simulink model "FourWheelSim_base"  (R2021b)
settings: Solver=ode4  StartTime=0.0  StopTime=100  FixedStep=0.001  EnableMultiTasking=on
values from neighbouring files (symbols this model uses):
  a_f = [1.434106444513048,-3.490394354141787e-04,2.761516722659314,6.000050177239062e+04,2.990012596710455e+03,-1.736376596503330e-04,0.526021936511837]    [VehicleParams20_ver230707.m]
  a_r = a_f    [VehicleParams20_ver230707.m]
  afx_f = [1.736519934348130,-2.903281841026900e-04,2.651682004580759,7.000047010028531e+04,3.270011055825476e+03,-0.001252141095807,1.596836353939939]    [VehicleParams20_ver230707.m]
  afx_r = afx_f    [VehicleParams20_ver230707.m]
  agx_f = [0.230000000000000,2.936116597489246e+04,7.137436879966481e+03,0,0]    [VehicleParams20_ver230707.m]
  agx_r = agx_f    [VehicleParams20_ver230707.m]
  agy_f = [0.852564208514954,3.000069064154418e+04,2.070023877794581e+03,-5.089267464508360e-04,0.519364283925805]    [VehicleParams20_ver230707.m]
  agy_r = agy_f    [VehicleParams20_ver230707.m]
  b_f = [3.436650779629654,1.566044221042620e-05,0.028598122547093,3.408741969645286e+03,5.995144285148312e+03,-1.736376595720277e-04,0.526021936449385]    [VehicleParams20_ver230707.m]
  Brake_Factor = 0.66    [VehicleParams20_ver230707.m]
  Cd = Cd/(40/3.6)^2    (= 0.6885)    [VehicleParams20_ver230707.m]
  CLF = DFf/40/40    (= 0.06)    [VehicleParams20_ver230707.m]
  CLR = DFr/40/40    (= 0.065)    [VehicleParams20_ver230707.m]
  cPiston_Area_F = 2*pi*(0.0254/2)^2    (= 0.00101341495819)    [VehicleParams20_ver230707.m]
  cPiston_Area_R = 2*pi*(0.0254/2)^2    (= 0.00101341495819)    [VehicleParams20_ver230707.m]
  delta = 15.5    [VehicleParams20_ver230707.m]
  df = 1.225    [VehicleParams20_ver230707.m]
  dr = 1.225    [VehicleParams20_ver230707.m]
  eff_Radius_F = (180/2-13.5)/1000    (= 0.0765)    [VehicleParams20_ver230707.m]
  eff_Radius_R = (180/2-13.5)/1000    (= 0.0765)    [VehicleParams20_ver230707.m]
  Fd = 60*2    (= 120)    [VehicleParams20_ver230707.m]
  Frtoe = 0    [VehicleParams20_ver230707.m]
  gear_f = 13.75    [VehicleParams20_ver230707.m]
  gear_r = 13.75    [VehicleParams20_ver230707.m]
  hg = 0.28    [VehicleParams20_ver230707.m]
  HV_voltage = 600    [VehicleParams20_ver230707.m]
  I = 112    [VehicleParams20_ver230707.m]
  ini_v = ini_speed/3.6    (= 10.4166666667)    [VehicleParams20_ver230707.m]
  Kframe = 5.94*10^6    (= 5940000)    [VehicleParams20_ver230707.m]
  kk_f = 2800*180/pi    (= 160428.182637)    [VehicleParams20_ver230707.m]
  kk_r = 4200*180/pi    (= 240642.273955)    [VehicleParams20_ver230707.m]
  krfr = 0.5    [VehicleParams20_ver230707.m]
  l = 1.530    (= 1.53)    [VehicleParams20_ver230707.m]
  lf = l*(1-WBf)    (= 0.7956)    [VehicleParams20_ver230707.m]
  lr = l*WBf    (= 0.7344)    [VehicleParams20_ver230707.m]
  M = 200+60    (= 260)    [VehicleParams20_ver230707.m]
  mu_tire_F = 0.587-0.587+0.55    (= 0.55)    [VehicleParams20_ver230707.m]
  mu_tire_R = 0.587-0.587+0.55    (= 0.55)    [VehicleParams20_ver230707.m]
  Mwf = Iwf/Rwf/Rwf    (= 3.82716814816)    [VehicleParams20_ver230707.m]
  Mwr = Iwr/Rwr/Rwr    (= 3.82716814816)    [VehicleParams20_ver230707.m]
  rcf = 0.000    (= 0)    [VehicleParams20_ver230707.m]
  rch = rcf*WBf+rcr*(1-WBf)    (= 0)    [VehicleParams20_ver230707.m]
  rcr = 0.000    (= 0)    [VehicleParams20_ver230707.m]
  Reartoe = -2    [VehicleParams20_ver230707.m]
  Rr_toe = Reartoe*pi/180    (= -0.0349065850399)    [VehicleParams20_ver230707.m]
  Rwf = 18*(25.4/1000)/2    (= 0.2286)    [VehicleParams20_ver230707.m]
  Rwr = 18*(25.4/1000)/2    (= 0.2286)    [VehicleParams20_ver230707.m]
  T_TireF = TireL_f/V    (= 0.036760000032)    [VehicleParams20_ver230707.m]
  T_TireR = TireL_r/V    (= 0.036760000032)    [VehicleParams20_ver230707.m]
  tspeed = 37.5    [VehicleParams20_ver230707.m]
  WBf = 0.48    [VehicleParams20_ver230707.m]
  zc_f = castrail_Fr/1000    (= 0)    [VehicleParams20_ver230707.m]
  zc_r = castrail_Rr/1000    (= 0)    [VehicleParams20_ver230707.m]
libraries: simulink x25, dspstat3 x1
(part 1 of 4)
settings Model: Creator=FEM  LastModifiedBy=tsuyoshi
settings SolverCC: ZeroCrossAlgorithm=Adaptive  AlgebraicLoopSolver=TrustRegion
settings DataIOCC: LimitDataPoints=on  SaveFormat=Array  ReturnWorkspaceOutputs=off
settings OptimizationCC: ExpressionDepthLimit=2147483647  LifeSpan=inf
settings DebuggingCC: UnderspecifiedInitializationDetection=Classic  MergeDetectMultiDrivingBlocksExec=none  MaxConsecutiveZCsMsg=none  SolverPrmCheckMsg=warning  StateNameClashWarn=warning  SFUnexpectedBacktrackingDiag=warning  SFNoUnconditionalDefaultTransitionDiag=warning  SFExecutionAtInitializationDiag=none  SFMachineParentedDataDiag=warning  ArithmeticOperatorsInVariantConditions=warning
settings HardwareCC: ProdBitPerPointer=32  ProdBitPerSizeT=32  ProdBitPerPtrDiffT=32  ProdLargestAtomicFloat=None  ProdIntDivRoundTo=Undefined  ProdEndianess=Unspecified  ProdWordSize=32  ProdHWDeviceType=32-bit Generic
settings ModelReferenceCC: PropagateSignalLabelsOutOfModel=off
settings SFSimCC: SimUseLocalCustomCode=off  CustomCodeUndefinedFunction=UseInterfaceOnly
settings RTWCC: RTWUseLocalCustomCode=off
settings CodeAppCC: StateflowObjectComments=on
settings GRTTargetCC: TargetLangStandard=C89/C90 (ANSI)
settings ConfigComp: CovMetricSettings=dw  CovSaveCumulativeToWorkspaceVar=on  CovSaveSingleToWorkspaceVar=on  CovExternalEMLEnable=off
settings SimscapeCC: SimscapeNormalizeSystem=off

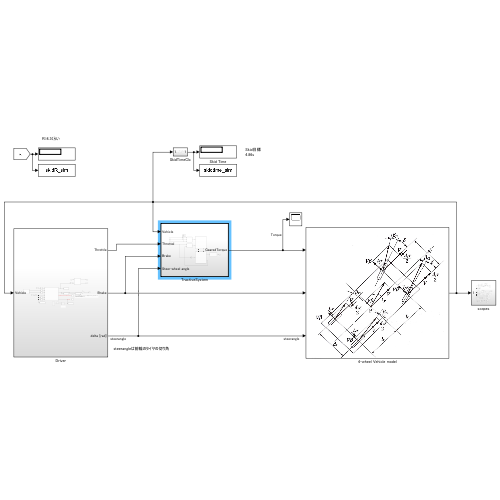
[thumbnail: Simulink's stored preview of the top-level diagram]
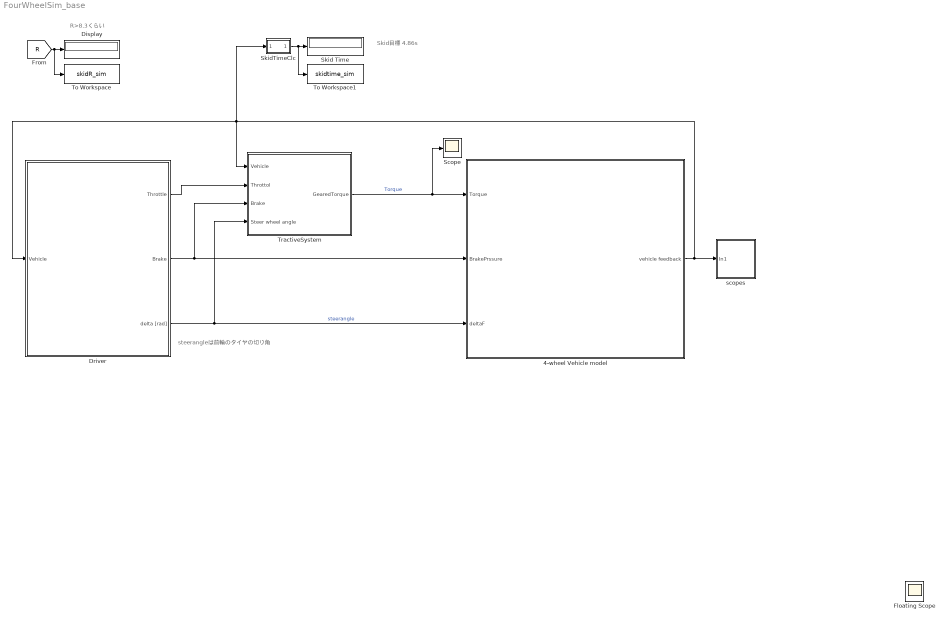
== system FourWheelSim_base ==
  note: R>8.3くらい
  note: Skid目標
      | 4.86s
  note: steerangleは前輪のタイヤの切り角
  4-wheel Vehicle model : Subsystem
      mask Display: image('$imagefile'); % 変更するには、ツールストリップの [イメージの編集] を使用してください。
  Display : Display
  Driver : Subsystem
  Scope : Scope
  Skid Time : Display
  SkidTimeClc : Subsystem
  To Workspace : ToWorkspace  VariableName=skidR_sim  SaveFormat=Timeseries  SampleTime=-1
  To Workspace1 : ToWorkspace  VariableName=skidtime_sim  SaveFormat=Timeseries  SampleTime=-1
  TractiveSystem : Subsystem  TreatAsAtomicUnit=on
  scopes : Subsystem
  Floating Scope : Scope
  wires:
  Driver/1(Throttle) -> TractiveSystem/2(Throttol)
  TractiveSystem/1(GearedTorque) -> 4-wheel Vehicle model/1(Torque), Scope/1  "Torque"
  4-wheel Vehicle model/1(vehicle feedback) -> SkidTimeClc/1(In1), Driver/1(Vehicle), TractiveSystem/1(Vehicle), scopes/1(In1)
  SkidTimeClc/1(Out1) -> To Workspace1/1, Skid Time/1
  [R] -> To Workspace/1, Display/1
  Driver/2(Brake) -> 4-wheel Vehicle model/2(BrakePrssure), TractiveSystem/3(Brake)
  Driver/3(delta [rad]) -> TractiveSystem/4(Steer wheel angle), 4-wheel Vehicle model/3(deltaF)  "steerangle"

== system FourWheelSim_base/4-wheel Vehicle model ==
  Torque : Inport
  BrakePrssure : Inport  Port=2
  deltaF : Inport  Port=3
  BrakeSystem : Subsystem
  Bus Creator2 : BusCreator  Inputs=4
  Constant : Constant  Value=Rr_toe
  Fin : Fcn  Expr=u+Frtoe*pi/180
  Fout : Fcn  Expr=u-Frtoe*pi/180
  Gain7 : Gain  Gain=-1
  comb slip model : Subsystem
      mask Display: image('$imagefile'); % 変更するには、ツールストリップの [イメージの編集] を使用してください。
  "equation of motion " : Subsystem
      mask Display: image('$imagefile'); % 変更するには、ツールストリップの [イメージの編集] を使用してください。
  force direction change : Subsystem
  to workspace : Subsystem
  vehicle feedback : Outport  VectorParamsAs1DForOutWhenUnconnected=off
  wires:
  Constant/1 -> Gain7/1, Bus Creator2/3  "delta_RL"
  comb slip model/1(tire force) -> force direction change/1(tire force)  "tire force"
  Bus Creator2/1 -> comb slip model/3(delta), force direction change/2(delta)  "delta"
  deltaF/1 -> Fin/1, Fout/1
  "equation of motion "/1(Vehicle Motion) -> to workspace/1(In1), comb slip model/1(Vehicle Motion)  "Vehicle Motion"
  Fout/1 -> Bus Creator2/2  "delta_FR"
  Fin/1 -> Bus Creator2/1  "delta_FL"
  Gain7/1 -> Bus Creator2/4  "delta_RR"
  Torque/1 -> BrakeSystem/2(GearedTorque)
  comb slip model/2(vehicle feedback) -> vehicle feedback/1
  force direction change/1(Long Force) -> "equation of motion "/1(Long Force)  "Long Force"
  force direction change/2(Yaw Moment) -> "equation of motion "/2(Yaw Moment)  "Yaw Moment"
  force direction change/3(Lat Force) -> "equation of motion "/3(Lat Force)  "Lat Force"
  BrakePrssure/1 -> BrakeSystem/1(BrakePrssure)
  BrakeSystem/1(NetTorque) -> comb slip model/2(Torque)

== system FourWheelSim_base/Driver ==
  note: 発散の原因
      | DYCゲイン過大：1
      | その他(トー過大?)：2
  note: Goto/Fromでつないだ場合，
      | 「Goto/From の接続は、非バーチャル サブシステムの境界をクロスできません。唯一の例外は、Goto が状態出力端子に接続される場合のみです」
      | エラーとなるのでForループを用いる．
  Vehicle : Inport
  Chart : Stateflow chart  TreatAsAtomicUnit=on
  Constant1 : Constant  Commented=on  Value=2
  Display : Display
  Gain1 : Gain  Gain=pi/180
  Memory{,1..3} (4 alike) : Memory
  Pylon Touch : Subsystem
  Saturation : Saturate  UpperLimit=200  LowerLimit=0
  SpeedControll : Subsystem
  Stop Simulation : Stop
  Stop Simulation1 : Stop
  Switch1 : Switch  Commented=on  Threshold=340*pi/360
  To Workspace1 : ToWorkspace  VariableName=Div  SaveFormat=Timeseries  SampleTime=-1
  To Workspace2 : ToWorkspace  VariableName=tspeed_sim  SaveFormat=Timeseries  SampleTime=-1
  To Workspace3 : ToWorkspace  VariableName=delta_sim  SaveFormat=Timeseries  SampleTime=-1
  To Workspace4 : ToWorkspace  VariableName=Vnow_sim  SaveFormat=Timeseries  SampleTime=-1
  Transport Delay : TransportDelay
  Transport Delay1 : TransportDelay  DelayTime=0.5
  βの最大変化量 : Subsystem  Commented=on
  Throttle : Outport
  Brake : Outport  Port=2
  delta [rad] : Outport  Port=3
  wires:
  Transport Delay/1 -> Chart/5(Vpre1)
  Pylon Touch/1(Rf) -> Memory1/1
  Pylon Touch/2(Rr) -> Memory2/1
  Chart/2(delta) -> To Workspace3/1, Gain1/1, Display/1
  [R] -> Memory/1
  Chart/3(Vopt) -> ?
  Chart/4(Div) -> To Workspace1/1
  Memory/1 -> Chart/1(R)
  Memory1/1 -> Chart/2(Rf)
  Memory2/1 -> Chart/3(Rr)
  [Vnow] -> Memory3/1
  Memory3/1 -> Transport Delay/1, To Workspace4/1, Transport Delay1/1, Chart/4(Vnow)
  Constant1/1 -> Switch1/1
  βの最大変化量/1(Outport) -> Switch1/2
  Transport Delay1/1 -> Chart/6(Vpre05)
  Saturation/1 -> SpeedControll/2(Target Speed)
  Chart/1(tspeed) -> Saturation/1, To Workspace2/1  "TargetSpeed(km/h)"
  Vehicle/1 -> SpeedControll/1(Vehicle speed)
  SpeedControll/1(Throttle) -> Throttle/1
  SpeedControll/2(Brake) -> Brake/1
  Gain1/1 -> delta [rad]/1  "deltaF(rad)"

== system FourWheelSim_base/SkidTimeClc ==
  In1 : Inport
  Bus Selector : BusSelector  OutputSignals=Vehicle Motion.Long Velocity
  Divide : Product  Inputs=*/
  Gain : Gain  Gain=2*pi
  m/s : Gain
  Out1 : Outport  VectorParamsAs1DForOutWhenUnconnected=off
  wires:
  m/s/1 -> Divide/2
  In1/1 -> Bus Selector/1
  [R] -> Gain/1
  Divide/1 -> Out1/1
  Gain/1 -> Divide/1
  Bus Selector/1 -> m/s/1  "<Long Velocity>"

== system FourWheelSim_base/TractiveSystem ==
  Vehicle : Inport
  Throttol : Inport  Port=2
  Brake : Inport  Port=3
  Steer wheel angle : Inport  Port=4
  AMK PowerUnit x4 : Subsystem
      settings: PortSchema="{\"entries\":[{\"content\":{\"sides\":[{\"content\":{\"connectorIds\":[\"In1\"]},\"type\":\"ConnectorPlacement.EquallySpacedRectSide\",\"uuid\":\"e990d11b-ff81-4335-9a22-6cdf713d4717\"},{\"content\":{\"connectorIds\":[\"Out1\",\"Out2\"],\"side\":\"RIGHT\"},\"type\":\"ConnectorPlacement.EquallySpacedRectSide\",\"uuid\":\"59e0e618-bfe7-45fe-904d-89bd6da9458c\"},{\"content\":{\"connectorIds\":[\"Out3\",\"In2\"],\"side\":\"TOP\"},\"type\":\"ConnectorPlacement.EquallySpacedRectSide\",\"uuid\":\"9e2b5955-7a03-4a6a-9f05-18476f3458b2\"}]},\"type\":\"ConnectorPlacement.EquallySpacedConnector\",\"uuid\":\"65fbb8fc-573a-4a64-b281-fb493310408d\"}],\"packageUris\":[\"http://schema.mathworks.com/mf0/Connector/R2020b\"],\"version\":\"1.0\"}"
  Bus Selector1 : BusSelector  OutputSignals=Wheel Speed
  Driver Input : Subsystem
  Gear : Subsystem
  Scope : Scope  NumInputPorts=3
  Sensors : Subsystem
  VCM : Subsystem
      settings: PortSchema="{\"entries\":[{\"content\":{\"sides\":[{\"content\":{\"connectorIds\":[\"In1\",\"In2\"]},\"type\":\"ConnectorPlacement.EquallySpacedRectSide\",\"uuid\":\"5e77dd93-b51c-479b-b5fe-6f6816a8f554\"},{\"content\":{\"connectorIds\":[],\"side\":\"RIGHT\"},\"type\":\"ConnectorPlacement.EquallySpacedRectSide\",\"uuid\":\"bf0d52ae-9b9e-4d5a-babc-26efa99ef7a4\"},{\"content\":{\"connectorIds\":[],\"side\":\"TOP\"},\"type\":\"ConnectorPlacement.EquallySpacedRectSide\",\"uuid\":\"b9d2ff59-7c1f-4a33-8b92-e641dfa19e52\"},{\"content\":{\"connectorIds\":[\"In3\",\"Out1\"],\"side\":\"BOTTOM\"},\"type\":\"ConnectorPlacement.EquallySpacedRectSide\",\"uuid\":\"e471c7ad-4e4d-4a43-b287-ecb0303bfc1b\"}]},\"type\":\"ConnectorPlacement.EquallySpacedConnector\",\"uuid\":\"5754af0f-8218-4685-b773-d9359332d734\"}],\"packageUris\":[\"http://schema.mathworks.com/mf0/Connector/R2020b\"],\"version\":\"1.0\"}"
  GearedTorque : Outport  VectorParamsAs1DForOutWhenUnconnected=off
  wires:
  Bus Selector1/1 -> AMK PowerUnit x4/1(Wheel speed)  "<Wheel Speed>"
  VCM/1(CAN out) -> AMK PowerUnit x4/2(CAN in)
  Driver Input/1(Driver Input) -> VCM/1(Driver in)
  AMK PowerUnit x4/3(CAN out) -> VCM/3(CAN in)
  Sensors/1(CAN to VCM) -> VCM/2(Sensor)
  AMK PowerUnit x4/2(Current) -> Sensors/2(Current)
  Throttol/1 -> Scope/1, Driver Input/1(Throttol)
  Vehicle/1 -> Bus Selector1/1, Sensors/1(Sensors)
  Steer wheel angle/1 -> Scope/3, Driver Input/3(Steer angle)
  Gear/1(GearedTorque) -> GearedTorque/1
  AMK PowerUnit x4/1(Motor trq) -> Gear/1(MotorTorque)
  Brake/1 -> Scope/2, Driver Input/2(Brake)

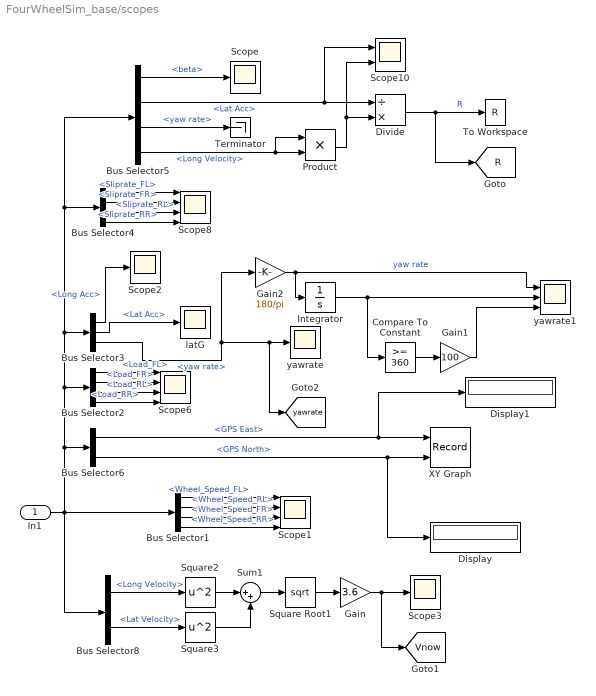
== system FourWheelSim_base/scopes ==
  In1 : Inport
  Bus Selector1 : BusSelector  OutputSignals=Wheel Speed.Wheel_Speed_FL,Wheel Speed.Wheel_Speed_RL,Wheel Speed.Wheel_Speed_FR,Wheel Speed.Wheel_Speed_RR
  Bus Selector2 : BusSelector  OutputSignals=tire status.load.Load_FL,tire status.load.Load_FR,tire status.load.Load_RL,tire status.load.Load_RR
  Bus Selector3 : BusSelector  OutputSignals=Vehicle Motion.Long Acc,Vehicle Motion.Lat Acc,Vehicle Motion.yaw rate
  Bus Selector4 : BusSelector  OutputSignals=tire status.Slip rate.Sliprate_FL,tire status.Slip rate.Sliprate_FR,tire status.Slip rate.Sliprate_RL,tire status.Slip rate.Sliprate_RR
  Bus Selector5 : BusSelector  OutputSignals=Vehicle Motion.beta,Vehicle Motion.Lat Acc,Vehicle Motion.yaw rate,Vehicle Motion.Long Velocity
  Bus Selector6 : BusSelector  OutputSignals=Vehicle Motion.GPS East,Vehicle Motion.GPS North
  Bus Selector8 : BusSelector  OutputSignals=Vehicle Motion.Long Velocity,Vehicle Motion.Lat Velocity
  Compare To Constant : simulink/Logic and Bit Operations/Compare To Constant  relop=>=  const=360  OutDataTypeStr=boolean
  Display : Display
  Display1 : Display
  Divide : Product  Inputs=/*
  Gain : Gain  Gain=3.6
  Gain1 : Gain  Gain=100
  Gain2 : Gain  Gain=180/pi
  Integrator : Integrator
  Product : Product
  Scope : Scope
  Scope1 : Scope  NumInputPorts=4
  Scope10 : Scope  NumInputPorts=2
  Scope2 : Scope
  Scope3 : Scope
  Scope6 : Scope  NumInputPorts=4
  Scope8 : Scope  NumInputPorts=4
  Square Root1 : Sqrt  SaturateOnIntegerOverflow=on
  Square2 : Math  Operator=square  SaturateOnIntegerOverflow=on
  Square3 : Math  Operator=square  SaturateOnIntegerOverflow=on
  Sum1 : Sum  Inputs=|++
  Terminator : Terminator
  To Workspace : ToWorkspace  VariableName=R  SaveFormat=Timeseries  SampleTime=-1
  XY Graph : Record  FileSettingsInternal="{\"entries\":[{\"content\":{\"excelSettings\":{\"content\":{},\"type\":\"Streamout.ExcelSettings\"}},\"type\":\"Streamout.FileSettingStorage\",\"uuid\":\"04da413e-0bc8-4522-bc77-97f7bd740fff\"}],\"packageUris\":[\"http://schema.mathworks.com/mf0/streamout_blocks/R2020a\"],\"version\":\"1.0\"}"  Layout=[1 1]  SignalsInternal="{\"entries\":[{\"content\":{\"signals\":[{\"content\":{\"blockPath\":[\"FourWheelSim_base/scopes/XY Graph\"],\"channel\":[],\"dimensions\":[1],\"domain\":\"FourWheelSim_base/scopes/XY Graph\",\"lineColor\":\"#77ac30\",\"plots\":[1],\"port\":1,\"sid\":[],\"signalID\":713,\"signalName\":\"<GPS East>\"},\"type\":\"RecordBlkView.Signal\",\"uuid\":\"76456aae-c6a4-477c-b0e6-9aa2acff60b4\"},{\"content\":{\"blockPath\":[\"FourWheelSim_base/scopes/XY Graph\"],\"channel\":[],\"dimensions\":[1],\"domain\":\"FourWheelSim_base/scopes/XY Graph\",\"lineColor\":\"#4dbeee\",\"plots\":[1],\"port\":2,\"sid\":[],\"signalID\":716,\"signalName\":\"<GPS North>\"},\"type\":\"RecordBlkView.Signal\",\"uuid\":\"c308d40b-e731-4fe8-a725-c3bc60c488fc\"}]},\"type\":\"RecordBlkView.InputSignals\",\"uuid\":\"f0e00ebc-5757-4aa9-ad1b-0663875eda47\"}],\"packageUris\":[\"http://schema.mathworks.com/mf0/streamout_blocks/R2020a\"],\"version\":\"1.0\"}"  VisualizationBindings="{\"xyplotplugin\":{\"info\":[{\"series\":[{\"bindingParametersList\":[{\"parameter\":\"X-Axis\",\"signalID\":713,\"signalName\":\"<GPS East>\"},{\"parameter\":\"Y-Axis\",\"signalID\":716,\"signalName\":\"<GPS North>\"}],\"seriesID\":50809}],\"subplotID\":1}]}}"  CompatibilityTag=XY  st=-1
  latG : Scope
  yawrate : Scope
  yawrate1 : Scope  NumInputPorts=3
  tag scope: R=global, Vnow=global, yawrate=global
  wires:
  Bus Selector3/2 -> latG/1  "<Lat Acc>"
  Compare To Constant/1 -> Gain1/1
  Bus Selector2/2 -> Scope6/2  "<Load_FR>"
  Gain2/1 -> Integrator/1, yawrate1/1  "yaw rate"
  Bus Selector5/1 -> Scope/1  "<beta>"
  Product/1 -> Divide/2, Scope10/2
  Divide/1 -> To Workspace/1, [R]  "R"
  Gain1/1 -> yawrate1/3
  Bus Selector4/1 -> Scope8/1  "<Sliprate_FL>"
  Bus Selector5/4 -> Product/1, Product/2  "<Long Velocity>"
  Bus Selector2/3 -> Scope6/3  "<Load_RL>"
  Bus Selector2/4 -> Scope6/4  "<Load_RR>"
  Bus Selector4/2 -> Scope8/2  "<Sliprate_FR>"
  Bus Selector4/3 -> Scope8/3  "<Sliprate_RL>"
  Bus Selector4/4 -> Scope8/4  "<Sliprate_RR>"
  Bus Selector3/3 -> [yawrate], yawrate/1, Gain2/1  "<yaw rate>"
  Bus Selector5/2 -> Scope10/1, Divide/1  "<Lat Acc>"
  Integrator/1 -> Compare To Constant/1, yawrate1/2
  Bus Selector2/1 -> Scope6/1  "<Load_FL>"
  Bus Selector5/3 -> Terminator/1  "<yaw rate>"
  Bus Selector1/1 -> Scope1/1  "<Wheel_Speed_FL>"
  Bus Selector1/2 -> Scope1/2  "<Wheel_Speed_RL>"
  Bus Selector1/3 -> Scope1/3  "<Wheel_Speed_FR>"
  Bus Selector1/4 -> Scope1/4  "<Wheel_Speed_RR>"
  Bus Selector6/1 -> Display1/1, XY Graph/1  "<GPS East>"
  Bus Selector6/2 -> Display/1, XY Graph/2  "<GPS North>"
  Square Root1/1 -> Gain/1
  Square3/1 -> Sum1/2
  Bus Selector8/2 -> Square3/1  "<Lat Velocity>"
  Bus Selector8/1 -> Square2/1  "<Long Velocity>"
  Square2/1 -> Sum1/1
  Gain/1 -> [Vnow], Scope3/1
  Sum1/1 -> Square Root1/1
  In1/1 -> Bus Selector8/1, Bus Selector6/1, Bus Selector5/1, Bus Selector4/1, Bus Selector3/1, Bus Selector2/1, Bus Selector1/1
  Bus Selector3/1 -> Scope2/1  "<Long Acc>"

== system FourWheelSim_base/4-wheel Vehicle model/BrakeSystem ==
  BrakePrssure : Inport
  GearedTorque : Inport  Port=2
  Add{,1..3} (4 alike) : Sum  Inputs=+-
  Bus Creator : BusCreator  Inputs=4
  Bus Selector : BusSelector  OutputSignals=FL,FR,RL,RR
  Gain2 : Gain  Gain=cPiston_Area_F*Brake_Factor*eff_Radius_F
  Gain4 : Gain  Gain=cPiston_Area_R*Brake_Factor*eff_Radius_R
  NetTorque : Outport  VectorParamsAs1DForOutWhenUnconnected=off
  wires:
  Bus Selector/2 -> Add1/1  "<FR>"
  Gain2/1 -> Add1/2, Add/2  "BrakeTorqueFr"
  Add2/1 -> Bus Creator/3  "RL"
  Add/1 -> Bus Creator/1  "FL"
  BrakePrssure/1 -> Gain4/1, Gain2/1
  Bus Selector/3 -> Add2/1  "<RL>"
  Bus Selector/1 -> Add/1  "<FL>"
  Bus Selector/4 -> Add3/1  "<RR>"
  Gain4/1 -> Add3/2, Add2/2  "BrakeTorqueRr"
  Bus Creator/1 -> NetTorque/1  "NetTorque"
  GearedTorque/1 -> Bus Selector/1
  Add1/1 -> Bus Creator/2  "FR"
  Add3/1 -> Bus Creator/4  "RR"

== system FourWheelSim_base/4-wheel Vehicle model/comb slip model ==
  Vehicle Motion : Inport
  Torque : Inport  Port=2
  delta : Inport  Port=3
  +MxLatG/framestiff : Subsystem
  +Mz : Subsystem
  Bus Creator1 : BusCreator  Inputs=3
  Bus Creator3 : BusCreator  Inputs=2
  Bus Creator4 : BusCreator  Inputs=3
  Load : Subsystem
      mask Display: image('$imagefile'); % 変更するには、ツールストリップの [イメージの編集] を使用してください。
  Mz calc : Subsystem
  Slip Angle : Subsystem
      mask Display: image('$imagefile'); % 変更するには、ツールストリップの [イメージの編集] を使用してください。
  Slip rate calc : Subsystem
      mask Display: image('$imagefile'); % 変更するには、ツールストリップの [イメージの編集] を使用してください。
  Wheel speed calc : Subsystem
      mask Display: image('$imagefile'); % 変更するには、ツールストリップの [イメージの編集] を使用してください。
  comb Fx calc : Subsystem
  comb Fy calc : Subsystem
  tire force : Outport  VectorParamsAs1DForOutWhenUnconnected=off
  vehicle feedback : Outport  Port=2  VectorParamsAs1DForOutWhenUnconnected=off
  wires:
  comb Fx calc/1(Fx) -> Bus Creator3/1  "Fx"
  comb Fy calc/1(Fy) -> Mz calc/1("Fy "), Bus Creator3/2  "Fy"
  Wheel speed calc/1(Wheel Speed) -> Bus Creator4/1, Slip rate calc/2(Wheel Speed)  "Wheel Speed"
  Load/1(Load) -> Bus Creator1/1  "load"
  Vehicle Motion/1 -> Bus Creator4/2, Load/1(Vehicle Motion), Slip rate calc/1(VehicleSpeed), Slip Angle/1(Vehicle Motion), +MxLatG/framestiff/1(Lat G)  "Vehicle Motion"
  +MxLatG/framestiff/1(delta2) -> Slip Angle/2(delta2)
  Bus Creator4/1 -> vehicle feedback/1
  Slip Angle/1(Slip_angle) -> Bus Creator1/3  "Slip angle"
  Slip rate calc/1("SlipRate ") -> Bus Creator1/2  "Slip rate"
  Bus Creator1/1 -> Mz calc/2(tire status), comb Fy calc/1(tire status), Bus Creator4/3, comb Fx calc/1(tire status)  "tire status"
  +Mz/1(delta1) -> +MxLatG/framestiff/2(delta1)
  Bus Creator3/1 -> Wheel speed calc/1(comb_Fx), tire force/1
  Torque/1 -> Wheel speed calc/2(Torque)
  Mz calc/1(Mz) -> +Mz/2(Mz)
  delta/1 -> +Mz/1(delta0)

== system FourWheelSim_base/4-wheel Vehicle model/equation of motion  ==
  Long Force : Inport
  Yaw Moment : Inport  Port=2
  Lat Force : Inport  Port=3
  Beta Angle : Subsystem
  Bus Creator1 : BusCreator  Inputs=11
  GPS cordinate Clc : Subsystem
  Net Long Force : Subsystem
  Roll Clc : Subsystem
  Yaw Clc : Subsystem
  equation of motion : Subsystem
  Vehicle Motion : Outport  VectorParamsAs1DForOutWhenUnconnected=off
  wires:
  Beta Angle/1(Body Beta Angle) -> Bus Creator1/9  "beta"
  Bus Creator1/1 -> Vehicle Motion/1
  GPS cordinate Clc/1(GPS East) -> Bus Creator1/5  "GPS East"
  GPS cordinate Clc/2(GPS North) -> Bus Creator1/6  "GPS North"
  Roll Clc/1(RollRate) -> Bus Creator1/10  "roll rate"
  Roll Clc/2(RollAngle) -> Bus Creator1/11  "roll angle"
  Yaw Clc/1(yaw rate) -> equation of motion/3(yaw rate), Bus Creator1/7  "yaw rate"
  Yaw Moment/1 -> Yaw Clc/1(Yaw Moment)
  Yaw Clc/2(yaw angle) -> GPS cordinate Clc/3(YawAngle), Bus Creator1/8  "yaw angle"
  equation of motion/4(Lat Velo) -> Beta Angle/1(Lat Velo), GPS cordinate Clc/2(Lat Velo), Bus Creator1/4  "Lat Velocity"
  equation of motion/2(Long Velo) -> GPS cordinate Clc/1(Long Velo), Beta Angle/2(Long Velo), Net Long Force/1(Vehicle speed), Bus Creator1/2  "Long Velocity"
  Long Force/1 -> Net Long Force/2(Long Force)
  equation of motion/1(Long Acc) -> Bus Creator1/1  "Long Acc"
  Net Long Force/1(Net Long Force) -> equation of motion/1(Net Long Force)  "Long Acc"
  Lat Force/1 -> equation of motion/2(Lat Force)  "Lat Force"
  equation of motion/3(Lat Acc) -> Roll Clc/1(Lat Acc), Bus Creator1/3  "Lat Acc"

== system FourWheelSim_base/4-wheel Vehicle model/force direction change ==
  tire force : Inport
  delta : Inport  Port=2
  Bus Creator1 : BusCreator  Inputs=3
  Bus Selector6 : BusSelector  OutputSignals=Fx,Fy
  Lat Force and Yaw Moment1 : Subsystem
  Long Force and Vectoring Yaw Moment : Subsystem
  Sum2 : Sum  Inputs=+|+
  sincos culc : Subsystem
  Long Force : Outport  VectorParamsAs1DForOutWhenUnconnected=off
  Yaw Moment : Outport  Port=2  VectorParamsAs1DForOutWhenUnconnected=off
  Lat Force : Outport  Port=3  VectorParamsAs1DForOutWhenUnconnected=off
  wires:
  Long Force and Vectoring Yaw Moment/2(Vectoring_Yaw_Moment) -> Sum2/1
  Long Force and Vectoring Yaw Moment/1(Long_Force) -> Long Force/1  "Long Force"
  Sum2/1 -> Yaw Moment/1  "Yaw Moment"
  Lat Force and Yaw Moment1/2(Lat_Force) -> Lat Force/1  "Lat Force"
  Lat Force and Yaw Moment1/1(Yaw_Moment) -> Sum2/2
  Bus Creator1/1 -> Lat Force and Yaw Moment1/1(In1), Long Force and Vectoring Yaw Moment/1(In1)
  Bus Selector6/2 -> Bus Creator1/2  "<Fy>"
  sincos culc/1(delta sincos) -> Bus Creator1/3  "delta sincos"
  Bus Selector6/1 -> Bus Creator1/1  "<Fx>"
  tire force/1 -> Bus Selector6/1
  delta/1 -> sincos culc/1(delta)  "delta"

== system FourWheelSim_base/4-wheel Vehicle model/to workspace ==
  In1 : Inport
  Bus Selector : BusSelector  OutputSignals=Long Acc,Long Velocity,beta,Lat Acc,yaw rate,GPS North,GPS East
  To Workspace : ToWorkspace  VariableName=Long_Acc  SaveFormat=Timeseries  SampleTime=-1
  To Workspace1 : ToWorkspace  VariableName=speed  SaveFormat=Timeseries  SampleTime=-1
  To Workspace2 : ToWorkspace  VariableName=beta  SaveFormat=Timeseries  SampleTime=-1
  To Workspace3 : ToWorkspace  VariableName=Lat_Acc  SaveFormat=Timeseries  SampleTime=-1
  To Workspace4 : ToWorkspace  VariableName=yawrate  SaveFormat=Timeseries  SampleTime=-1
  To Workspace5 : ToWorkspace  VariableName=X  SampleTime=-1
  To Workspace6 : ToWorkspace  VariableName=Y  SampleTime=-1
  wires:
  In1/1 -> Bus Selector/1
  Bus Selector/1 -> To Workspace/1  "<Long Acc>"
  Bus Selector/2 -> To Workspace1/1  "<Long Velocity>"
  Bus Selector/3 -> To Workspace2/1  "<beta>"
  Bus Selector/4 -> To Workspace3/1  "<Lat Acc>"
  Bus Selector/5 -> To Workspace4/1  "<yaw rate>"
  Bus Selector/6 -> To Workspace6/1  "<GPS North>"
  Bus Selector/7 -> To Workspace5/1  "<GPS East>"

== system FourWheelSim_base/Driver/Pylon Touch ==
  R : Subsystem
  Scope : Scope  NumInputPorts=3
  Square : Math  Operator=square  SaturateOnIntegerOverflow=on
  Square Root : Sqrt  SaturateOnIntegerOverflow=on
  Square Root1 : Sqrt  SaturateOnIntegerOverflow=on
  Square1 : Math  Operator=square  SaturateOnIntegerOverflow=on
  Sum : Sum  Inputs=+++
  Sum1 : Sum  Inputs=+++
  Sum2 : Sum  Inputs=+
  Sum3 : Sum  Inputs=+
  rt : Subsystem
  rw : Subsystem
  Rf : Outport
  Rr : Outport  Port=2
  wires:
  rw/1(rwf) -> Sum/2  "rwf"
  rw/2(rwr) -> Sum1/2  "rwr"
  R/1(R) -> Sum/1, Sum1/1  "R"
  rt/1(rtf) -> Sum/3  "rtf"
  rt/2(rtr) -> Sum1/3  "rtr"
  Sum/1 -> Square1/1
  Sum1/1 -> Square/1
  Square/1 -> Sum3/1
  Square1/1 -> Sum2/1
  Sum2/1 -> Square Root/1
  Sum3/1 -> Square Root1/1
  Square Root/1 -> Rf/1, Scope/2  "Rf"
  Square Root1/1 -> Rr/1, Scope/3  "Rr"
  [R] -> Scope/1

== system FourWheelSim_base/Driver/SpeedControll ==
  note: 車両のスピードをPID制御してるブロック
  Vehicle speed : Inport
  Target Speed : Inport  Port=2
  Add : Sum  Inputs=+-
  Add1 : Sum  Inputs=+++
  Bus Selector : BusSelector  OutputSignals=Vehicle Motion.Long Velocity
  DGain : Gain  Gain=0.5
  Gain : Gain  Gain=-1
  Gain1 : Gain  Gain=1/10
  Gain2 : Gain  Gain=100
  Gain22 : Gain  Gain=3.6
  IGain : Gain  Gain=2
  PGain : Gain  Gain=3
  Saturation : Saturate  UpperLimit=1  LowerLimit=0
  Saturation1 : Saturate  UpperLimit=5  LowerLimit=0
  Scope : Scope
  Scope5 : Scope  NumInputPorts=2
  TargetSpeed : Constant  Commented=on  Value=tspeed
  Transfer Fcn : TransferFcn  Numerator=[1 0]  Denominator=[0.01 1]
  sekibun : Integrator  LowerSaturationLimit=0
  Throttle : Outport  VectorParamsAs1DForOutWhenUnconnected=off
  Brake : Outport  Port=2  VectorParamsAs1DForOutWhenUnconnected=off
  tag scope: TargetSpeed=global
  wires:
  Add/1 -> Gain1/1
  PGain/1 -> Add1/1
  sekibun/1 -> Add1/2
  DGain/1 -> Transfer Fcn/1
  Vehicle speed/1 -> Bus Selector/1
  Gain22/1 -> Scope5/2, Add/2  "Speed[km/h]"
  Bus Selector/1 -> Gain22/1  "<Long Velocity>"
  Target Speed/1 -> [TargetSpeed], Add/1, Scope5/1  "Target Speed"
  Saturation/1 -> Throttle/1  "Throttle"
  IGain/1 -> sekibun/1
  Saturation1/1 -> Gain2/1  "Brake"
  Gain/1 -> Saturation1/1
  Add1/1 -> Scope/1, Gain/1, Saturation/1
  Transfer Fcn/1 -> Add1/3
  Gain1/1 -> DGain/1, IGain/1, PGain/1
  Gain2/1 -> Brake/1  "BrakePressure"

== system FourWheelSim_base/Driver/βの最大変化量 ==
  Abs : Abs
  Constant : Constant  Value=0
  Memory4 : Memory
  Memory5 : Memory
  MinMax Running Resettable : simulink/Math Operations/MinMax Running Resettable  Function=max  vinit=0.0
  Sum : Sum  Inputs=|+-
  Outport : Outport
  wires:
  Memory5/1 -> Sum/2
  Sum/1 -> Abs/1
  Abs/1 -> MinMax Running Resettable/1
  [B] -> Memory4/1
  Constant/1 -> MinMax Running Resettable/2
  MinMax Running Resettable/1 -> Outport/1
  Memory4/1 -> Sum/1, Memory5/1

== system FourWheelSim_base/TractiveSystem/AMK PowerUnit x4 ==
  note: FEM20
      | 番号タイヤ対応表
      | 1:FR 2:RR
      | 3:RL 4:FL
  Wheel speed : Inport
  CAN in : Inport  Port=2
  All Power consumption : Subsystem
  Bus Creator : BusCreator  Inputs=4
  Bus Selector : BusSelector  OutputSignals=Wheel_Speed_FR,Wheel_Speed_RR,Wheel_Speed_RL,Wheel_Speed_FL
  CAN from Inv : Subsystem
  Discrete FIR Filter : DiscreteFir  Coefficients=[0.1 0.1 0.1 0.1 0.1 0.1 0.1 0.1 0.1 0.1]
  Divide : Product  Inputs=*/
  Gain : Gain  Gain=gear_f*60/(2*Rwf*pi)
  Gain1 : Gain  Gain=gear_r*60/(2*Rwf*pi)
  Gain2 : Gain  Gain=gear_f*60/(2*Rwf*pi)
  Gain3 : Gain  Gain=gear_r*60/(2*Rwr*pi)
  HV_voltage : Constant  Value=HV_voltage
  HV_voltage1 : Constant  Value=HV_voltage
  INV dummy : Subsystem
  Moving Average : dspstat3/Moving Average  Method=Sliding window  ForgettingFactorPort=off  SpecifyWindowLength=on  WindowLength=500  ForgettingFactor=0.9  SimulateUsing=Code generation
  Scope{1..4} (4 alike) : Scope
  Motor trq : Outport  VectorParamsAs1DForOutWhenUnconnected=off
  Current : Outport  Port=2  VectorParamsAs1DForOutWhenUnconnected=off
  CAN out : Outport  Port=3  VectorParamsAs1DForOutWhenUnconnected=off
  wires:
  INV dummy/6(MC_33) -> CAN from Inv/6(In6)
  INV dummy/14(Motor2_Trq) -> Bus Creator/2  "RR Torque"
  INV dummy/13(Motor1_Trq) -> Bus Creator/1  "FR Torque"
  INV dummy/1(MC_11) -> CAN from Inv/1(In1)
  INV dummy/2(MC_12) -> CAN from Inv/2(In2)
  INV dummy/5(MC_32) -> CAN from Inv/5(In5)
  INV dummy/9(MC_23) -> CAN from Inv/9(In9)
  HV_voltage/1 -> INV dummy/1(HV_DC)
  INV dummy/10(MC_41) -> CAN from Inv/10(In10)
  INV dummy/4(MC_31) -> CAN from Inv/4(In4)
  INV dummy/11(MC_42) -> CAN from Inv/11(In11)
  Gain1/1 -> INV dummy/4(Motor2_RPM)
  INV dummy/3(MC_13) -> CAN from Inv/3(In3)
  INV dummy/7(MC_21) -> CAN from Inv/7(In7)
  Gain/1 -> INV dummy/3(Motor1_RPM)
  INV dummy/12(MC_43) -> CAN from Inv/12(In12)
  INV dummy/8(MC_22) -> CAN from Inv/8(In8)
  CAN in/1 -> INV dummy/2(CAN to Inv)
  CAN from Inv/1(CAN from Inv) -> CAN out/1
  Divide/1 -> Current/1
  Discrete FIR Filter/1 -> Scope1/1
  Moving Average/1 -> Scope2/1
  Gain3/1 -> INV dummy/5(Motor3_RPM)
  Gain2/1 -> INV dummy/6(Motor4_RPM)
  INV dummy/15(Motor3_Trq) -> Bus Creator/3  "RL Torque"
  INV dummy/16(Motor4_Trq) -> Bus Creator/4  "FL Torque"
  Bus Creator/1 -> Scope4/1, Motor trq/1, All Power consumption/1(Motor trq)  "Motor trq"
  Wheel speed/1 -> All Power consumption/2(Wheel speed), Scope3/1, Bus Selector/1
  HV_voltage1/1 -> Divide/2
  Bus Selector/1 -> Gain/1  "<Wheel_Speed_FR>"
  Bus Selector/2 -> Gain1/1  "<Wheel_Speed_RR>"
  Bus Selector/3 -> Gain3/1  "<Wheel_Speed_RL>"
  Bus Selector/4 -> Gain2/1  "<Wheel_Speed_FL>"
  All Power consumption/1(All Power consumption [W]) -> Moving Average/1, Divide/1, Discrete FIR Filter/1

== system FourWheelSim_base/TractiveSystem/Driver Input ==
  Throttol : Inport
  Brake : Inport  Port=2
  Steer angle : Inport  Port=3
  Bus Creator : BusCreator  Inputs=10
  Compare To Zero : simulink/Logic and Bit Operations/Compare To Zero  relop=>  OutDataTypeStr=boolean
  Constant1 : Constant
  Delay : Delay  DelayLength=1
  Error Reset Switch1 : Constant  Value=0
  Gain : Gain
  Gain2 : Gain
  Launch Switch : Constant  Value=0
  PedalForce to Pressure : Subsystem  ReferencedSubsystem=PedalForce_to_Pressure
  Ready to Drive Switch : Constant  Value=0
  Driver Input : Outport  VectorParamsAs1DForOutWhenUnconnected=off
  wires:
  Error Reset Switch1/1 -> Bus Creator/9  "ErrorResetSW"
  Ready to Drive Switch/1 -> Bus Creator/7  "RtoDSW"
  Throttol/1 -> Delay/1
  Steer angle/1 -> Gain2/1
  Gain2/1 -> Bus Creator/2  "SteerAngle_Actual"
  Bus Creator/1 -> Driver Input/1  "Driver Input"
  Constant1/1 -> Bus Creator/10  "VDCSW"
  Launch Switch/1 -> Bus Creator/8  "LaunchSW"
  Delay/1 -> Bus Creator/1  "APPS Actual"
  Compare To Zero/1 -> Bus Creator/6  "Brake SW"
  Gain/1 -> Bus Creator/5  "BrakePressF_Calibrated"
  PedalForce to Pressure/2 -> Gain/1, Bus Creator/4  "BrakePressR"
  PedalForce to Pressure/1 -> Bus Creator/3  "BrakePressF"
  Brake/1 -> PedalForce to Pressure/1, Compare To Zero/1  "Brake Pedal Force"

== system FourWheelSim_base/TractiveSystem/Gear ==
  note: 将来的にギアの特性入れれるといいかもね
  MotorTorque : Inport
  Bus Creator1 : BusCreator  Inputs=4
  Bus Selector2 : BusSelector  OutputSignals=FL Torque,RL Torque,FR Torque,RR Torque
  Gain1 : Gain  Gain=gear_f
  Gain2 : Gain  Gain=gear_f
  Gain3 : Gain  Gain=gear_r
  Gain4 : Gain  Gain=gear_r
  GearedTorque : Outport  VectorParamsAs1DForOutWhenUnconnected=off
  wires:
  Gain1/1 -> Bus Creator1/1  "FL"
  MotorTorque/1 -> Bus Selector2/1
  Gain2/1 -> Bus Creator1/3  "FR"
  Bus Creator1/1 -> GearedTorque/1  "GearedTorque"
  Gain4/1 -> Bus Creator1/4  "RR"
  Bus Selector2/2 -> Gain3/1  "<RL Torque>"
  Bus Selector2/3 -> Gain2/1  "<FR Torque>"
  Gain3/1 -> Bus Creator1/2  "RL"
  Bus Selector2/4 -> Gain4/1  "<RR Torque>"
  Bus Selector2/1 -> Gain1/1  "<FL Torque>"

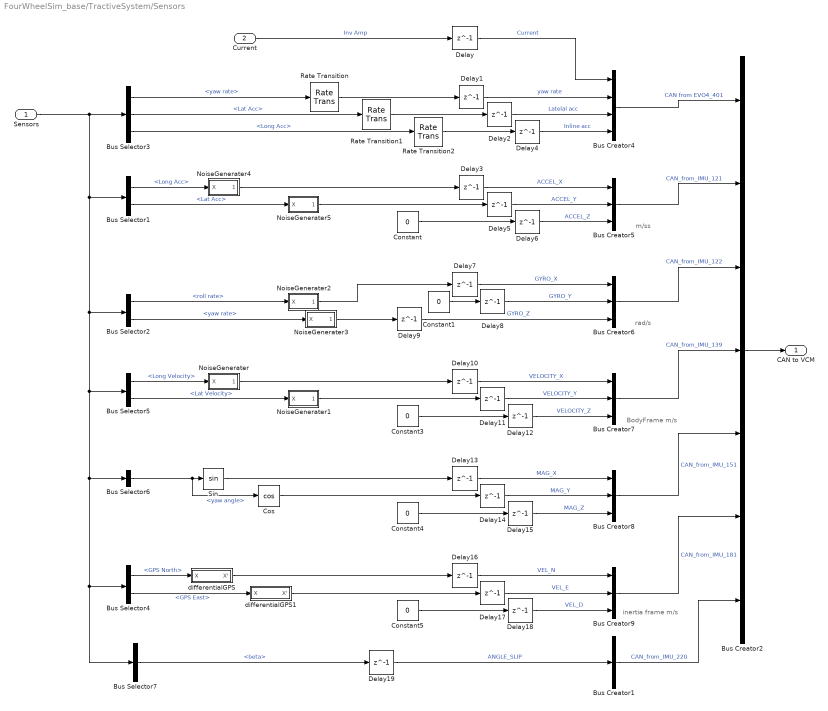
== system FourWheelSim_base/TractiveSystem/Sensors ==
  note: inertia frame
      | m/s
  note: m/ss
  note: rad/s
  note: BodyFrame
      | m/s
  Sensors : Inport
  Current : Inport  Port=2
  Bus Creator1 : BusCreator  Inputs=1
  Bus Creator2 : BusCreator  Inputs=7
  Bus Creator4 : BusCreator  Inputs=4
  Bus Creator{5..9} (5 alike) : BusCreator  Inputs=3
  Bus Selector1 : BusSelector  OutputSignals=Vehicle Motion.Long Acc,Vehicle Motion.Lat Acc
  Bus Selector2 : BusSelector  OutputSignals=Vehicle Motion.roll rate,Vehicle Motion.yaw rate
  Bus Selector3 : BusSelector  OutputSignals=Vehicle Motion.yaw rate,Vehicle Motion.Lat Acc,Vehicle Motion.Long Acc
  Bus Selector4 : BusSelector  OutputSignals=Vehicle Motion.GPS North,Vehicle Motion.GPS East
  Bus Selector5 : BusSelector  OutputSignals=Vehicle Motion.Long Velocity,Vehicle Motion.Lat Velocity
  Bus Selector6 : BusSelector  OutputSignals=Vehicle Motion.yaw angle
  Bus Selector7 : BusSelector  OutputSignals=Vehicle Motion.beta
  Constant{,1,3..5} (5 alike) : Constant  Value=0
  Cos : Trigonometry  Operator=cos
  Delay{,1..19} (20 alike) : Delay  DelayLength=1
  NoiseGenerater : Subsystem
  NoiseGenerater1 : Subsystem
  NoiseGenerater2 : Subsystem
  NoiseGenerater3 : Subsystem
  NoiseGenerater4 : Subsystem
  NoiseGenerater5 : Subsystem
  Rate Transition : RateTransition  OutPortSampleTime=0.02
  Rate Transition1 : RateTransition  OutPortSampleTime=0.02
  Rate Transition2 : RateTransition  OutPortSampleTime=0.02
  Sin : Trigonometry
  differentialGPS : Subsystem
  differentialGPS1 : Subsystem
  CAN to VCM : Outport  VectorParamsAs1DForOutWhenUnconnected=off
  wires:
  Current/1 -> Delay/1  "Inv Amp"
  Delay/1 -> Bus Creator4/1  "Current"
  Delay13/1 -> Bus Creator8/1  "MAG_X"
  Bus Creator9/1 -> Bus Creator2/6  "CAN_from_IMU_181"
  Bus Creator6/1 -> Bus Creator2/3  "CAN_from_IMU_122"
  Delay4/1 -> Bus Creator4/4  "Inline acc"
  Delay1/1 -> Bus Creator4/2  "yaw rate"
  Delay10/1 -> Bus Creator7/1  "VELOCITY_X"
  Delay17/1 -> Bus Creator9/2  "VEL_E"
  Delay16/1 -> Bus Creator9/1  "VEL_N"
  Delay18/1 -> Bus Creator9/3  "VEL_D"
  Bus Creator8/1 -> Bus Creator2/5  "CAN_from_IMU_151"
  Delay12/1 -> Bus Creator7/3  "VELOCITY_Z"
  Delay7/1 -> Bus Creator6/1  "GYRO_X"
  Delay8/1 -> Bus Creator6/2  "GYRO_Y"
  Bus Creator5/1 -> Bus Creator2/2  "CAN_from_IMU_121"
  Delay11/1 -> Bus Creator7/2  "VELOCITY_Y"
  Delay14/1 -> Bus Creator8/2  "MAG_Y"
  Bus Creator4/1 -> Bus Creator2/1  "CAN from EVO4_401"
  Delay15/1 -> Bus Creator8/3  "MAG_Z"
  Bus Creator7/1 -> Bus Creator2/4  "CAN_from_IMU_139"
  Delay9/1 -> Bus Creator6/3  "GYRO_Z"
  Bus Creator2/1 -> CAN to VCM/1
  Delay2/1 -> Bus Creator4/3  "Latelal acc"
  Bus Selector3/3 -> Rate Transition2/1  "<Long Acc>"
  Bus Selector3/1 -> Rate Transition/1  "<yaw rate>"
  Bus Selector3/2 -> Rate Transition1/1  "<Lat Acc>"
  NoiseGenerater2/1(X+X') -> Delay7/1
  Bus Selector2/1 -> NoiseGenerater2/1(X)  "<roll rate>"
  Bus Selector2/2 -> NoiseGenerater3/1(X)  "<yaw rate>"
  Constant3/1 -> Delay12/1
  Constant4/1 -> Delay15/1
  Constant5/1 -> Delay18/1
  Bus Selector4/1 -> differentialGPS/1(X)  "<GPS North>"
  Bus Selector4/2 -> differentialGPS1/1(X)  "<GPS East>"
  differentialGPS/1(X') -> Delay16/1
  differentialGPS1/1(X') -> Delay17/1
  Bus Selector5/2 -> NoiseGenerater1/1(X)  "<Lat Velocity>"
  Bus Selector5/1 -> NoiseGenerater/1(X)  "<Long Velocity>"
  Bus Selector6/1 -> Sin/1, Cos/1  "<yaw angle>"
  Sin/1 -> Delay13/1
  Cos/1 -> Delay14/1
  NoiseGenerater/1(X+X') -> Delay10/1
  NoiseGenerater1/1(X+X') -> Delay11/1
  NoiseGenerater3/1(X+X') -> Delay9/1
  Rate Transition/1 -> Delay1/1
  Rate Transition1/1 -> Delay2/1
  Rate Transition2/1 -> Delay4/1
  Sensors/1 -> Bus Selector1/1, Bus Selector5/1, Bus Selector6/1, Bus Selector7/1, Bus Selector4/1, Bus Selector2/1, Bus Selector3/1
  Bus Selector1/1 -> NoiseGenerater4/1(X)  "<Long Acc>"
  NoiseGenerater5/1(X+X') -> Delay5/1
  Constant/1 -> Delay6/1
  NoiseGenerater4/1(X+X') -> Delay3/1
  Delay3/1 -> Bus Creator5/1  "ACCEL_X"
  Delay6/1 -> Bus Creator5/3  "ACCEL_Z"
  Delay5/1 -> Bus Creator5/2  "ACCEL_Y"
  Bus Selector1/2 -> NoiseGenerater5/1(X)  "<Lat Acc>"
  Bus Selector7/1 -> Delay19/1  "<beta>"
  Delay19/1 -> Bus Creator1/1  "ANGLE_SLIP"
  Bus Creator1/1 -> Bus Creator2/7  "CAN_from_IMU_220"
  Constant1/1 -> Delay8/1

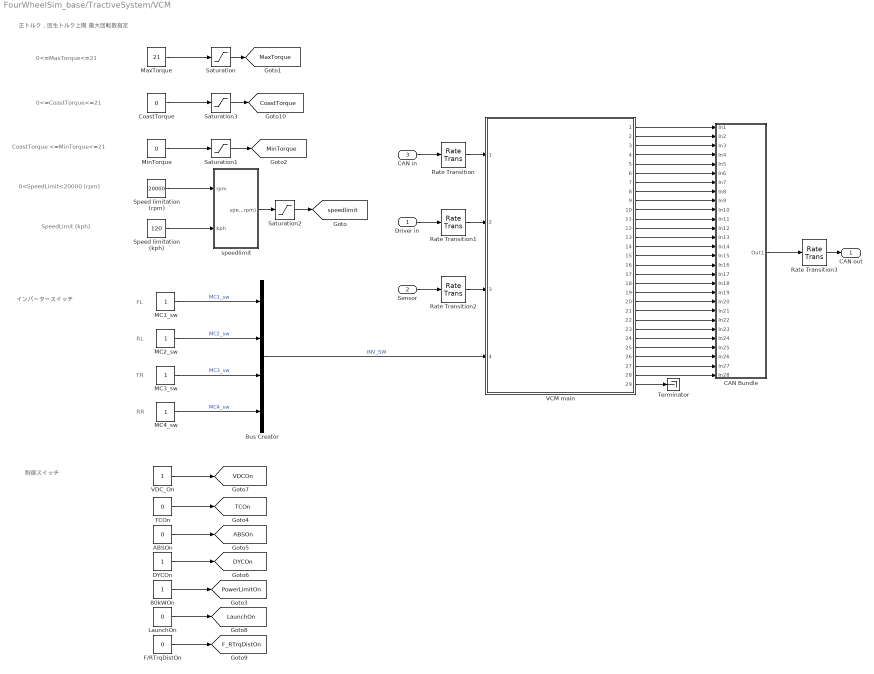
== system FourWheelSim_base/TractiveSystem/VCM ==
  note: FL
  note: FR
  note: CoastTorque <=MinTorque<=21
  note: RL
  note: SpeedLimit (kph)
  note: インバータースイッチ
  note: 制御スイッチ
  note: 正トルク，回生トルク上限
      | 最大回転数指定
  note: RR
  note: 0<=CoastTorque<=21
  note: 0<=MaxTorque<=21
  note: 0<SpeedLimit<20000 (rpm)
  Driver in : Inport
  Sensor : Inport  Port=2
  CAN in : Inport  Port=3
  80kWOn : Constant
  ABSOn : Constant  Value=0
  Bus Creator : BusCreator  Inputs=4
  CAN Bundle : Subsystem
  CoastTorque : Constant  Value=0
  DYCOn : Constant
  F/RTrqDistOn : Constant  Value=0
  LaunchOn : Constant  Value=0
  MC1_sw : Constant
  MC2_sw : Constant
  MC3_sw : Constant
  MC4_sw : Constant
  MaxTorque : Constant  Value=21
  MinTorque : Constant  Value=0
  Rate Transition : RateTransition  OutPortSampleTime=0.001
  Rate Transition1 : RateTransition  OutPortSampleTime=0.001
  Rate Transition2 : RateTransition  OutPortSampleTime=0.001
  Rate Transition3 : RateTransition
  Saturation : Saturate  UpperLimit=21  LowerLimit=0
  Saturation1 : Saturate  UpperLimit=21  LowerLimit=0
  Saturation2 : Saturate  UpperLimit=19500  LowerLimit=0
  Saturation3 : Saturate  UpperLimit=21  LowerLimit=0
  Speed limitation (kph) : Constant  Value=120
  Speed limitation (rpm) : Constant  Value=20000
  TCOn : Constant  Value=0
  Terminator : Terminator
  VCM main : Subsystem  ReferencedSubsystem=VCM_main_ver3_0_0
  VDC_On : Constant
  speedlimit : Subsystem
  CAN out : Outport  VectorParamsAs1DForOutWhenUnconnected=off
  tag scope: ABSOn=global, CoastTorque=global, DYCOn=global, F_RTrqDistOn=global, LaunchOn=global, MaxTorque=global, MinTorque=global, PowerLimitOn=global, TCOn=global, VDCOn=global, speedlimit=global
  wires:
  Saturation3/1 -> [CoastTorque]
  VCM main/28 -> CAN Bundle/28(In28)
  MinTorque/1 -> Saturation1/1
  Speed limitation (rpm)/1 -> speedlimit/1(rpm)
  VCM main/8 -> CAN Bundle/8(In8)
  CAN in/1 -> Rate Transition/1
  TCOn/1 -> [TCOn]
  Saturation1/1 -> [MinTorque]
  Bus Creator/1 -> VCM main/4  "INV_SW"
  VCM main/29 -> Terminator/1
  MC2_sw/1 -> Bus Creator/2  "MC2_sw"
  LaunchOn/1 -> [LaunchOn]
  Speed limitation (kph)/1 -> speedlimit/2(kph)
  VCM main/23 -> CAN Bundle/23(In23)
  VCM main/7 -> CAN Bundle/7(In7)
  MC3_sw/1 -> Bus Creator/3  "MC3_sw"
  VCM main/26 -> CAN Bundle/26(In26)
  speedlimit/1(speedlimit(rpm)) -> Saturation2/1
  VCM main/12 -> CAN Bundle/12(In12)
  VCM main/1 -> CAN Bundle/1(In1)
  CAN Bundle/1(Out1) -> Rate Transition3/1
  VCM main/25 -> CAN Bundle/25(In25)
  Saturation/1 -> [MaxTorque]
  VCM main/20 -> CAN Bundle/20(In20)
  VCM main/15 -> CAN Bundle/15(In15)
  MaxTorque/1 -> Saturation/1
  ABSOn/1 -> [ABSOn]
  VCM main/2 -> CAN Bundle/2(In2)
  VDC_On/1 -> [VDCOn]
  Driver in/1 -> Rate Transition1/1
  VCM main/10 -> CAN Bundle/10(In10)
  MC4_sw/1 -> Bus Creator/4  "MC4_sw"
  VCM main/6 -> CAN Bundle/6(In6)
  DYCOn/1 -> [DYCOn]
  MC1_sw/1 -> Bus Creator/1  "MC1_sw"
  VCM main/19 -> CAN Bundle/19(In19)
  80kWOn/1 -> [PowerLimitOn]
  VCM main/11 -> CAN Bundle/11(In11)
  VCM main/22 -> CAN Bundle/22(In22)
  VCM main/9 -> CAN Bundle/9(In9)
  VCM main/5 -> CAN Bundle/5(In5)
  VCM main/4 -> CAN Bundle/4(In4)
  VCM main/14 -> CAN Bundle/14(In14)
  VCM main/17 -> CAN Bundle/17(In17)
  VCM main/21 -> CAN Bundle/21(In21)
  VCM main/3 -> CAN Bundle/3(In3)
  VCM main/18 -> CAN Bundle/18(In18)
  VCM main/13 -> CAN Bundle/13(In13)
  VCM main/24 -> CAN Bundle/24(In24)
  Sensor/1 -> Rate Transition2/1
  CoastTorque/1 -> Saturation3/1
  F/RTrqDistOn/1 -> [F_RTrqDistOn]
  VCM main/27 -> CAN Bundle/27(In27)
  VCM main/16 -> CAN Bundle/16(In16)
  Saturation2/1 -> [speedlimit]
  Rate Transition/1 -> VCM main/1
  Rate Transition1/1 -> VCM main/2
  Rate Transition2/1 -> VCM main/3
  Rate Transition3/1 -> CAN out/1

== system FourWheelSim_base/4-wheel Vehicle model/comb slip model/+MxLatG//framestiff ==
  Lat G : Inport
  delta1 : Inport  Port=2
  Bus Creator : BusCreator  Inputs=4
  Bus Selector : BusSelector  OutputSignals=delta_FL,delta_FR,delta_RL,delta_RR
  Bus Selector1 : BusSelector  OutputSignals=Lat Acc
  Display : Display
  Frame Stiff : Gain  Gain=M/Kframe
  Sum{5..8} (4 alike) : Sum  Inputs=|++
  delta2 : Outport  VectorParamsAs1DForOutWhenUnconnected=off
  wires:
  delta1/1 -> Bus Selector/1
  Bus Selector/4 -> Sum8/1  "<delta_RR>"
  Bus Selector/3 -> Sum7/1  "<delta_RL>"
  Bus Selector/2 -> Sum6/1  "<delta_FR>"
  Bus Selector/1 -> Sum5/1  "<delta_FL>"
  Sum5/1 -> Bus Creator/1  "delta_FL"
  Sum6/1 -> Bus Creator/2  "delta_FR"
  Sum7/1 -> Bus Creator/3  "delta_RL"
  Sum8/1 -> Bus Creator/4  "delta_RR"
  Bus Creator/1 -> delta2/1
  Frame Stiff/1 -> Sum6/2, Sum5/2, Sum7/2, Sum8/2
  Lat G/1 -> Bus Selector1/1
  Bus Selector1/1 -> Display/1, Frame Stiff/1  "<Lat Acc>"

== system FourWheelSim_base/4-wheel Vehicle model/comb slip model/+Mz ==
  delta0 : Inport
  Mz : Inport  Port=2
  Bus Creator : BusCreator  Inputs=4
  Bus Selector : BusSelector  OutputSignals=delta_FL,delta_FR,delta_RL,delta_RR
  Bus Selector1 : BusSelector  OutputSignals=MZ_FL,MZ_FR,MZ_RL,MZ_RR
  Sum{5..8} (4 alike) : Sum  Inputs=|++
  delta1 : Outport  VectorParamsAs1DForOutWhenUnconnected=off
  wires:
  delta0/1 -> Bus Selector/1
  Bus Selector/4 -> Sum8/1  "<delta_RR>"
  Bus Selector/3 -> Sum7/1  "<delta_RL>"
  Bus Selector/2 -> Sum6/1  "<delta_FR>"
  Bus Selector/1 -> Sum5/1  "<delta_FL>"
  Sum5/1 -> Bus Creator/1  "delta_FL"
  Sum6/1 -> Bus Creator/2  "delta_FR"
  Sum7/1 -> Bus Creator/3  "delta_RL"
  Sum8/1 -> Bus Creator/4  "delta_RR"
  Bus Creator/1 -> delta1/1
  Mz/1 -> Bus Selector1/1
  Bus Selector1/1 -> Sum5/2  "<MZ_FL>"
  Bus Selector1/2 -> Sum6/2  "<MZ_FR>"
  Bus Selector1/3 -> Sum7/2  "<MZ_RL>"
  Bus Selector1/4 -> Sum8/2  "<MZ_RR>"

== system FourWheelSim_base/4-wheel Vehicle model/comb slip model/Load ==
  Vehicle Motion : Inport
  Add{,4..5,7..9} (6 alike) : Sum
  Add3 : Sum  Inputs=+-
  Add6 : Sum  Inputs=-+
  Bus Creator : BusCreator  Inputs=4
  Bus Selector : BusSelector  OutputSignals=Long Acc,Lat Acc,Long Velocity
  FR Load Diff : Subsystem  ReferencedSubsystem=FR_Load_Diff
  Front DF : Gain  Gain=CLF/2
  Gain : Gain  Gain=3.6
  Product : Product
  RL Load Diff : Subsystem
  Rear DF : Gain  Gain=CLR/2
  Load : Outport  VectorParamsAs1DForOutWhenUnconnected=off
  wires:
  Add5/1 -> Bus Creator/2  "Load_FR"
  Add/1 -> Bus Creator/1  "Load_FL"
  Add8/1 -> Bus Creator/3  "Load_RL"
  Add9/1 -> Bus Creator/4  "Load_RR"
  Bus Selector/3 -> Gain/1  "<Long Velocity>"
  Product/1 -> Rear DF/1, Front DF/1
  Front DF/1 -> Add/2, Add5/2
  Rear DF/1 -> Add8/2, Add9/2
  Bus Creator/1 -> Load/1
  Vehicle Motion/1 -> Bus Selector/1
  RL Load Diff/2(Rear Load Diff_RL) -> Add6/1, Add7/1
  RL Load Diff/1(Front Load Diff_RL) -> Add3/2, Add4/2
  Bus Selector/2 -> RL Load Diff/3(LatG)  "<Lat Acc>"
  Add3/1 -> Add/1
  Add4/1 -> Add5/1
  Add6/1 -> Add8/1
  Add7/1 -> Add9/1
  Gain/1 -> Product/2, Product/1  "Long velo [km/h]"
  FR Load Diff/1 -> RL Load Diff/1(FrontLoad), Add4/1, Add3/1
  FR Load Diff/2 -> Add6/2, Add7/2, RL Load Diff/2(RearLoad)
  Bus Selector/1 -> FR Load Diff/1  "<Long Acc>"

== system FourWheelSim_base/4-wheel Vehicle model/comb slip model/Mz calc ==
  note: アライニングトルクの式らしい
  "Fy " : Inport
  tire status : Inport  Port=2
  Add{,1..3} (4 alike) : Sum
  Bus Creator : BusCreator  Inputs=4
  Bus Selector : BusSelector  OutputSignals=load.Load_FL,Slip angle.SA_FL,Slip rate.Sliprate_FL
  Bus Selector1 : BusSelector  OutputSignals=load.Load_FR,Slip angle.SA_FR,Slip rate.Sliprate_FR
  Bus Selector2 : BusSelector  OutputSignals=load.Load_RL,Slip angle.SA_RL,Slip rate.Sliprate_RL
  Bus Selector3 : BusSelector  OutputSignals=load.Load_RR,Slip angle.SA_RR,Slip rate.Sliprate_RR
  Bus Selector4 : BusSelector  OutputSignals=Fy_FL,Fy_FR,Fy_RL,Fy_RR
  Gain10 : Gain  Gain=-zc_r
  Gain11 : Gain  Gain=-zc_r
  Gain12 : Gain  Gain=1/kk_f
  Gain13 : Gain  Gain=1/kk_f
  Gain14 : Gain  Gain=1/kk_r
  Gain15 : Gain  Gain=1/kk_r
  Gain8 : Gain  Gain=-zc_f
  Gain9 : Gain  Gain=-zc_f
  MZ sw : Constant  Value=0
  MZ_Fin : Subsystem
  MZ_Fout : Subsystem
  MZ_Rin : Subsystem
  MZ_Rout : Subsystem
  Product{,1..3} (4 alike) : Product
  Mz : Outport  VectorParamsAs1DForOutWhenUnconnected=off
  wires:
  Gain11/1 -> Add3/1
  Gain9/1 -> Add1/1
  Gain10/1 -> Add2/1
  Gain8/1 -> Add/1
  MZ_Fin/1(MZ_Fin) -> Add/2
  MZ_Fout/1(MZ_Fin) -> Add1/2
  MZ_Rin/1(MZ_Fin) -> Add2/2
  MZ_Rout/1(MZ_Fin) -> Add3/2
  Add/1 -> Product/1
  Product/1 -> Gain12/1
  Add1/1 -> Product1/1
  Product1/1 -> Gain13/1
  Add2/1 -> Product2/1
  Product2/1 -> Gain14/1
  Add3/1 -> Product3/1
  Product3/1 -> Gain15/1
  MZ sw/1 -> Product3/2, Product2/2, Product1/2, Product/2
  Bus Selector1/2 -> MZ_Fout/2(beta_Fin)  "<SA_FR>"
  Bus Selector1/3 -> MZ_Fout/3(delta_Fin)  "<Sliprate_FR>"
  tire status/1 -> Bus Selector/1, Bus Selector3/1, Bus Selector2/1, Bus Selector1/1
  Bus Selector/2 -> MZ_Fin/2(beta_Fin)  "<SA_FL>"
  Bus Selector1/1 -> MZ_Fout/1(W_Fin)  "<Load_FR>"
  Bus Selector/3 -> MZ_Fin/3(delta_Fin)  "<Sliprate_FL>"
  Bus Selector/1 -> MZ_Fin/1(W_Fin)  "<Load_FL>"
  Bus Selector2/1 -> MZ_Rin/1(W_Fin)  "<Load_RL>"
  Bus Selector2/2 -> MZ_Rin/2(beta_Fin)  "<SA_RL>"
  Bus Selector2/3 -> MZ_Rin/3(delta_Fin)  "<Sliprate_RL>"
  Bus Selector3/1 -> MZ_Rout/1(W_Fin)  "<Load_RR>"
  Bus Selector3/2 -> MZ_Rout/2(beta_Fin)  "<SA_RR>"
  Bus Selector3/3 -> MZ_Rout/3(delta_Fin)  "<Sliprate_RR>"
  Gain12/1 -> Bus Creator/1  "MZ_FL"
  Gain13/1 -> Bus Creator/2  "MZ_FR"
  Gain14/1 -> Bus Creator/3  "MZ_RL"
  Gain15/1 -> Bus Creator/4  "MZ_RR"
  Bus Creator/1 -> Mz/1
  "Fy "/1 -> Bus Selector4/1
  Bus Selector4/1 -> Gain8/1  "<Fy_FL>"
  Bus Selector4/2 -> Gain9/1  "<Fy_FR>"
  Bus Selector4/3 -> Gain10/1  "<Fy_RL>"
  Bus Selector4/4 -> Gain11/1  "<Fy_RR>"
